simulink model "EDoS_model"  (R2020b)
settings: Solver=VariableStepAuto  StartTime=0.0  StopTime=200000  RelTol=1e-3
values from neighbouring files (symbols this model uses):
  attackRate = 0    [init_model.m]
  initialLoopWaitTime = 1000    [init_model.m]    (also in plot_results.m = 50)
  lowerUtilThreshold = 50    [init_model.m]    (also in plot_results.m)
  maxCores = 35    [init_model.m]    (also in plot_results.m)
  routineRate = 4    [init_model.m]    (also in plot_results.m)
  scalingLoopDelay = 500    [init_model.m]    (also in plot_results.m = 5)
  scalingStep = 2    [init_model.m]    (also in plot_results.m)
  upperUtilThreshold = 80    [init_model.m]    (also in plot_results.m)
undefined symbols (not defined in the file or in its folder): m, n
libraries: simulink x2
(part 1 of 3)
settings Model: Creator=evgen  LastModifiedBy=evgen

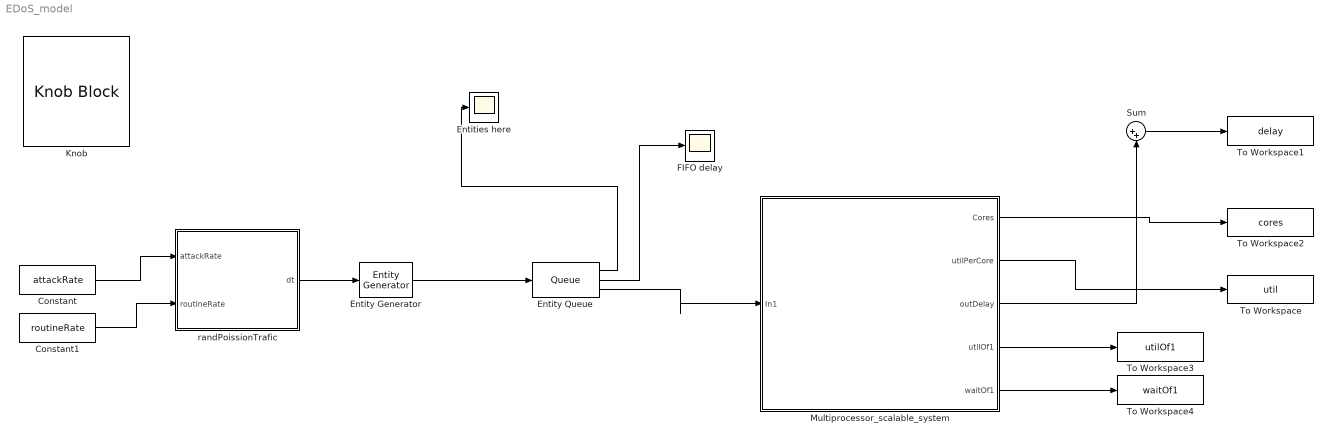
== system EDoS_model ==
  Constant : Constant  Value=attackRate  SampleTime=1
  Constant1 : Constant  Value=routineRate  SampleTime=1
  Entities here : Scope
  Entity Generator : EntityGenerator  OutputPortMessageModes=m  TimeSource=Signal port  IntergenerationTimeAction=|  AttributeName=ServiceTime  AttributeInitialValue=3  EntityType=Structured  EntityTypeName=Entity
      | lambda = 10;
      |     c = 0.767 - 3.36/lambda;
      |     beta = pi/sqrt(3.0*lambda);
      |     alpha = beta*lambda;
      |     k = log(c) - lambda - log(beta);
      | 
      |     while true
      |         u = rand(1);
      | 	    x = (alpha - log((1.0 - u)/u))/beta;
      | 	    n = floor(x + 0.5);
      | 	    if (n < 0)
      | 		    continue;
      |         end    
      | 	    v = rand(1);
      | 	    y = alpha - beta*x;
      | 	    lhs = y + log(v/(1.0 + exp(y))^2);
      | 	    rhs = k + n*log(lambda) - log(factorial(n));
      | 	    if (lhs <= rhs)
      | 		    break;
      |         end    
      |     end  
      |     dt = n/10;
      settings: InputPortMap=u1
  Entity Queue : Queue  InputPortMessageModes=m  OutputPortMessageModes=n,n,m  Capacity=10  NumberEntitiesInBlock=on  AverageWait=on
      settings: OutputPortMap=o1,o2,o5
  FIFO delay : Scope
  Knob : KnobBlock  ScaleMax=20
  Multiprocessor_scalable_system : Subsystem
  Sum : Sum  Inputs=|++
  To Workspace : ToWorkspace  VariableName=util  SaveFormat=Timeseries  SampleTime=-1
  To Workspace1 : ToWorkspace  VariableName=delay  SaveFormat=Timeseries  SampleTime=-1
  To Workspace2 : ToWorkspace  VariableName=cores  SaveFormat=Timeseries  SampleTime=-1
  To Workspace3 : ToWorkspace  VariableName=utilOf1  SaveFormat=Timeseries  SampleTime=-1
  To Workspace4 : ToWorkspace  VariableName=waitOf1  SaveFormat=Timeseries  SampleTime=-1
  randPoissionTrafic : MATLAB Function  TreatAsAtomicUnit=on
  wires:
  Entity Generator/1 -> Entity Queue/1
  Entity Queue/2 -> FIFO delay/1
  Entity Queue/3 -> Multiprocessor_scalable_system/1(In1)
  Multiprocessor_scalable_system/1(Cores) -> To Workspace2/1
  Multiprocessor_scalable_system/2(utilPerCore) -> To Workspace/1
  randPoissionTrafic/1(dt) -> Entity Generator/1
  Constant/1 -> randPoissionTrafic/1(attackRate)
  Constant1/1 -> randPoissionTrafic/2(routineRate)
  Entity Queue/1 -> Entities here/1
  Sum/1 -> To Workspace1/1
  Multiprocessor_scalable_system/3(outDelay) -> Sum/2
  Multiprocessor_scalable_system/4(utilOf1) -> To Workspace3/1
  Multiprocessor_scalable_system/5(waitOf1) -> To Workspace4/1
